simulink model "bh_boat_stabilizer_model"  (R2022b)
settings: Solver=ode15s  StartTime=0.0  StopTime=45  RelTol=1e-6  AbsTol=1e-6  EnableMultiTasking=on
undefined symbols (not defined in the file or in its folder): cage, disk, hull, my_points, sigbuilder_block, stand, X, Y, Z
libraries: sm_lib x37, nesl_utility x18, simulink_extras x18, simulink x1
(part 1 of 3)
settings Model: Creator=bhorton  LastModifiedBy=bhorton
settings SolverCC: ZeroCrossAlgorithm=Adaptive  AlgebraicLoopSolver=TrustRegion
settings DataIOCC: LimitDataPoints=on  MaxDataPoints=10000
settings OptimizationCC: LifeSpan=inf
settings DebuggingCC: UnconnectedInputMsg=warning  UnconnectedOutputMsg=warning  UnconnectedLineMsg=warning  AllowSymbolicDim=off  SFUnexpectedBacktrackingDiag=warning  SFNoUnconditionalDefaultTransitionDiag=warning  SFExecutionAtInitializationDiag=none  SFMachineParentedDataDiag=warning  ArithmeticOperatorsInVariantConditions=warning
settings ModelReferenceCC: EnableRefExpFcnMdlSchedulingChecks=on
settings SFSimCC: SimUseLocalCustomCode=off  CustomCodeUndefinedFunction=UseInterfaceOnly
settings RTWCC: RTWUseLocalCustomCode=off  DLArmComputeVersion=19.05
settings CodeAppCC: StateflowObjectComments=on
settings GRTTargetCC: TargetLangStandard=C89/C90 (ANSI)
settings ConfigComp: CovMetricSettings=dw  CovSaveCumulativeToWorkspaceVar=on  CovSaveSingleToWorkspaceVar=on  CovExternalEMLEnable=off  CovSFcnEnable=off
settings SimscapeCC: SimscapeLogType=all  SimscapeLogSimulationStatistics=on  SimscapeLogDataHistory=10000
settings ExplorerConfigSet: InternalSimMechanicsExplorerSettings="<ExplorerConfiguration><canonicalview>default</canonicalview><AnimationSetting><BasePlaybackSpeed>1.0</BasePlaybackSpeed><PlaybackSpeedFactor>1.0</PlaybackSpeedFactor></AnimationSetting><TilePanel><TileInfo><Tiles Columns=\"2\" Count=\"3\" Rows=\"2\"><Column Weight=\"0.5\"/><Column Weight=\"0.5\"/><Row Weight=\"0.4994\"/><Row Weight=\"0.5006\"/><Tile Height=\"2\" Width=\"1\" X=\"0\" Y=\"0\"/><Tile Height=\"1\" Width=\"1\" X=\"1\" Y=\"0\"/><Tile Height=\"1\" Width=\"1\" X=\"1\" Y=\"1\"/></Tiles></TileInfo><SceneInfo><SceneViewer><BGColor><R>0.60000002384185791</R><G>0.60000002384185791</G><B>0.60000002384185791</B></BGColor><Camera><DoPerspective>off</DoPerspective><Position><X>2.72907980115163751</X><Y>1.63827710737355892</Y><Z>5.84466597133086818</Z></Position><Center><X>1.48957165804863778</X><Y>-0.312477395456248752</Y><Z>2.71114995707715156</Z></Center><Up><X>0.0871556787867786148</X><Y>0.8298702872998307</Y><Z>-0.551107243567087735</Z></Up><ViewLimDist>1</ViewLimDist><YLim>5.28419304463390116</YLim><XLim>3.96508464876347055</XLim></Camera></SceneViewer><SceneViewer><BGColor><R>0.60000002384185791</R><G>0.60000002384185791</G><B>0.60000002384185791</B></BGColor><Camera><DoPerspective>off</DoPerspective><Position><X>0.174100554176560618</X><Y>2.79843990503689621</Y><Z>0.284823193336330216</Z></Position><Center><X>0.177652103694306729</X><Y>-0.924710698878394188</Y><Z>0.283383219246318929</Z></Center><Up><X>0.00583965905908712894</X><Y>0.000392326129121878253</Y><Z>-0.999982872084458463</Z></Up><ViewLimDist>1</ViewLimDist><YLim>0.869664947050413972</YLim><XLim>1.32261544030583789</XLim></Camera></SceneViewer><SceneViewer><BGColor><R>0.60000002384185791</R><G>0.60000002384185791</G><B>0.60000002384185791</B></BGColor><Camera><DoPerspective>off</DoPerspective><Position><X>-0.273643330341835023</X><Y>-1.00050075945724948</Y><Z>3.47750989252231513</Z></Position><Center><X>-0.273643330341835023</X><Y>-1.00050075945724948</Y><Z>-3.69061607941034708e-08</Z></Center><Up><X>0</X><Y>1</Y><Z>-0</Z></Up><ViewLimDist>1</ViewLimDist><YLim>2.77031267511226043</YLim><XLim>4.21318386006656276</XLim></Camera></SceneViewer></SceneInfo></TilePanel><MechEditorPanel><Cameras/><GfxPanelCameraMap/><VideoCreator><PlaybackSpeedRatio>1.0</PlaybackSpeedRatio><FrameRate>30</FrameRate><VideoFormat>Motion JPEG AVI</VideoFormat><FrameSize>auto</FrameSize></VideoCreator></MechEditorPanel></ExplorerConfiguration>"

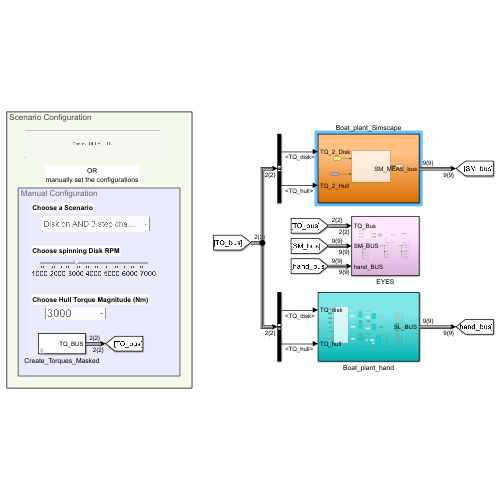
[thumbnail: Simulink's stored preview of the top-level diagram]
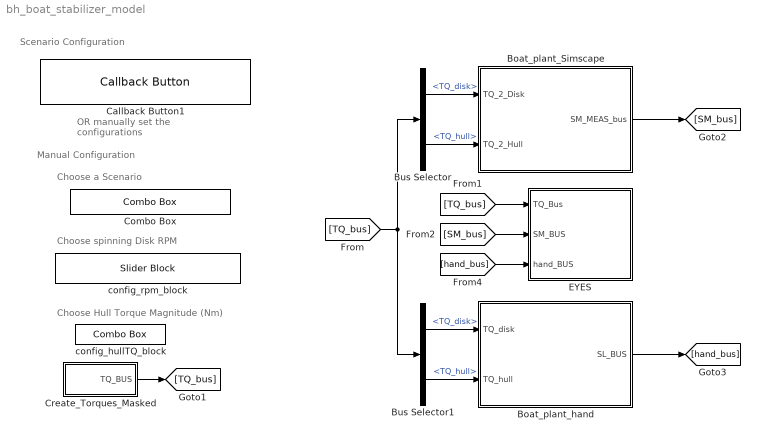
== system bh_boat_stabilizer_model ==
  note: Scenario Configuration
  note: OR
      | manually set the configurations
  note: Choose a Scenario
  note: Manual Configuration
  note: Choose spinning Disk RPM
  note: Choose Hull Torque Magnitude (Nm)
  Boat_plant_Simscape : Subsystem
  Boat_plant_hand : Subsystem
  Bus Selector : BusSelector  OutputSignals=TQ_disk,TQ_hull
  Bus Selector1 : BusSelector  OutputSignals=TQ_disk,TQ_hull
  Callback Button1 : CallbackButton  ButtonText=Choose DEFAULTS
      settings: ClickFcn=|
      | THE_BLOCK = [bdroot, '/Create_Torques_Masked'];
      | 
      | set_param(THE_BLOCK,'the_scenario','1');
      | set_param(THE_BLOCK,'the_disk_rpm','3000');
      | set_param(THE_BLOCK,'the_tau_hull','3000');
  Combo Box : ComboBox  LabelPosition=Hide  SelectedLabel=Disk on AND 3 step changes
      settings: Values={{'NO Stabilization (disk is NOT spinning)', 'Spin up disk BEFORE Disturbance', 'Spin up disk AFTER disturbance', 'Disk always spinning', 'Disk on AND 3 step changes', 'Spin Ramp to 10 percent'}, [1 2 3 4 5 6]}
  Create_Torques_Masked : Subsystem  mask{the_scenario=5, the_disk_rpm=3025.477707006369, the_tau_hull=3000}
      mask prompts: the_scenario "Scenario ID"; the_disk_rpm "Disk RPM"; the_tau_hull "Magnitude of HULL torque (N.m)"
      mask init:
      | THE_BLOCK = [gcb,'/my_sig_builder'];
      | signalbuilder(THE_BLOCK,'activegroup',the_scenario)
  EYES : Subsystem
  config_hullTQ_block : ComboBox  LabelPosition=Hide  SelectedLabel=3000
      settings: Values={{'1000', '3000', '5000', '7000', '9000', '11000'}, [1000 3000 5000 7000 9000 11000]}
  config_rpm_block : SliderBlock  LabelPosition=Hide  ScaleMin=1000  ScaleMax=7000  TickInterval=1000
  wires:
  Bus Selector/1 -> Boat_plant_Simscape/1(TQ_2_Disk)  "<TQ_disk>"
  Bus Selector/2 -> Boat_plant_Simscape/2(TQ_2_Hull)  "<TQ_hull>"
  Boat_plant_Simscape/1(SM_MEAS_bus) -> [SM_bus]
  [SM_bus] -> EYES/2(SM_BUS)
  [TQ_bus] -> EYES/1(TQ_Bus)
  Boat_plant_hand/1(SL_BUS) -> [hand_bus]
  [TQ_bus] -> Bus Selector1/1, Bus Selector/1
  [hand_bus] -> EYES/3(hand_BUS)
  Create_Torques_Masked/1(TQ_BUS) -> [TQ_bus]
  Bus Selector1/1 -> Boat_plant_hand/1(TQ_disk)  "<TQ_disk>"
  Bus Selector1/2 -> Boat_plant_hand/2(TQ_hull)  "<TQ_hull>"

== system bh_boat_stabilizer_model/Boat_plant_Simscape ==
  TQ_2_Disk : Inport
  TQ_2_Hull : Inport  Port=2
  Boat_SM : Subsystem
  SM_MEAS_bus : Outport
  wires:
  TQ_2_Disk/1 -> Boat_SM/1(TQ_spin_disk)
  Boat_SM/1(SM_MEAS_bus) -> SM_MEAS_bus/1
  TQ_2_Hull/1 -> Boat_SM/2(TQ_2_Hull)

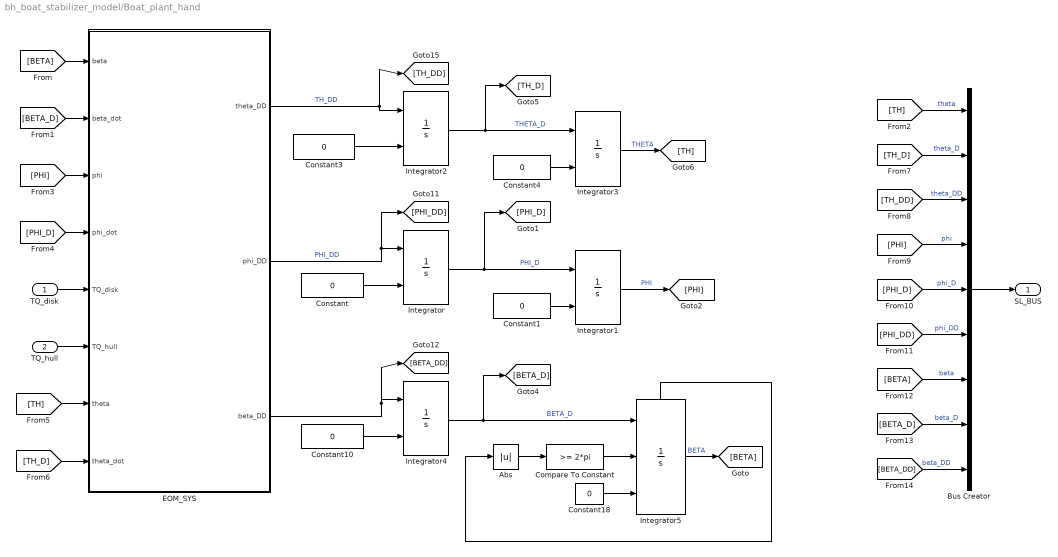
== system bh_boat_stabilizer_model/Boat_plant_hand ==
  TQ_disk : Inport
  TQ_hull : Inport  Port=2
  Abs : Abs  SaturateOnIntegerOverflow=off
  Bus Creator : BusCreator  Inputs=9
  Compare To Constant : simulink/Logic and Bit Operations/Compare To Constant  relop=>=  const=2*pi  OutDataTypeStr=boolean
  Constant{,1,3..4,10,18} (6 alike) : Constant  Value=0
  EOM_SYS : Subsystem
  Integrator{,1..4} (5 alike) : Integrator  InitialConditionSource=external
  Integrator5 : Integrator  ExternalReset=either  InitialConditionSource=external  ShowStatePort=on  AbsoluteTolerance=1e-8
  SL_BUS : Outport
  wires:
  Integrator3/1 -> [TH]  "THETA"
  Integrator4/1 -> [BETA_D], Integrator5/1  "BETA_D"
  Constant4/1 -> Integrator3/2
  Integrator2/1 -> [TH_D], Integrator3/1  "THETA_D"
  Integrator/1 -> [PHI_D], Integrator1/1  "PHI_D"
  Constant18/1 -> Integrator5/3
  Constant1/1 -> Integrator1/2
  Constant10/1 -> Integrator4/2
  Integrator1/1 -> [PHI]  "PHI"
  Constant/1 -> Integrator/2
  Constant3/1 -> Integrator2/2
  Integrator5/1 -> [BETA]  "BETA"
  EOM_SYS/1(theta_DD) -> [TH_DD], Integrator2/1  "TH_DD"
  EOM_SYS/2(phi_DD) -> [PHI_DD], Integrator/1  "PHI_DD"
  EOM_SYS/3(beta_DD) -> [BETA_DD], Integrator4/1
  TQ_disk/1 -> EOM_SYS/5(TQ_disk)
  TQ_hull/1 -> EOM_SYS/6(TQ_hull)
  [BETA_D] -> EOM_SYS/2(beta_dot)
  [BETA] -> EOM_SYS/1(beta)
  [TH_D] -> EOM_SYS/8(theta_dot)
  [TH] -> EOM_SYS/7(theta)
  [PHI_D] -> EOM_SYS/4(phi_dot)
  [PHI] -> EOM_SYS/3(phi)
  Bus Creator/1 -> SL_BUS/1
  [TH] -> Bus Creator/1  "theta"
  [TH_D] -> Bus Creator/2  "theta_D"
  [TH_DD] -> Bus Creator/3  "theta_DD"
  [PHI] -> Bus Creator/4  "phi"
  [PHI_D] -> Bus Creator/5  "phi_D"
  [PHI_DD] -> Bus Creator/6  "phi_DD"
  [BETA_DD] -> Bus Creator/9  "beta_DD"
  [BETA_D] -> Bus Creator/8  "beta_D"
  [BETA] -> Bus Creator/7  "beta"
  Abs/1 -> Compare To Constant/1
  Compare To Constant/1 -> Integrator5/2
  Integrator5/State -> Abs/1

== system bh_boat_stabilizer_model/Create_Torques_Masked ==
  Bus Creator : BusCreator  Inputs=2
  Create_DISK_w_TQ : Subsystem
  Enabled Subsystem1 : Subsystem  TreatAsAtomicUnit=on
  my_sig_builder : Subsystem  Tag=STV Subsys  LoadFcn=sigbuilder_block('load');  StartFcn=sigbuilder_block('start');  StopFcn=sigbuilder_block('stop');  ClipboardFcn=sigbuilder_block('clipboard');  mask(Sigbuilder block){tuvar=[0:10]}
      mask help: Simulink:masks:SigbuilderBlock_MD
      mask init:
      | if ~strcmp(get_param(bdroot(gcbh),'SimulationStatus'),'stopped') tuvar = sigbuilder_block('maskInit'); end
      settings: CopyFcn=sigbuilder_block('copy');  DeleteFcn=sigbuilder_block('delete');  ModelCloseFcn=sigbuilder_block('modelClose');  PreSaveFcn=sigbuilder_block('preSave');  PauseFcn=sigbuilder_block('pause');  ContinueFcn=sigbuilder_block('continue');  NameChangeFcn=sigbuilder_block('namechange');  OpenFcn=sigbuilder_block('open',[437.6 199.2 550.4 400 ]);  CloseFcn=sigbuilder_block('close');
      mask Display: plot(0, 0, 100, 100,[2, 2, 32, 32, 2], [68, 8, 8, 68, 68],[32, 2], [38, 38], [32, 19, 2],[53, 60, 44], [32, 17, 17, 2],[16, 16, 31, 31]);txt = getActiveGroup(gcbh);text(2, 100, txt,'verticalAlignment', 'top');
  TQ_BUS : Outport
  wires:
  my_sig_builder/1(DISK) -> Create_DISK_w_TQ/1(w_disk_normalised)
  Create_DISK_w_TQ/1(TQ) -> Bus Creator/1  "TQ_disk"
  Enabled Subsystem1/1(Out1) -> Bus Creator/2  "TQ_hull"
  my_sig_builder/2(HULL) -> Enabled Subsystem1/Enable
  Bus Creator/1 -> TQ_BUS/1

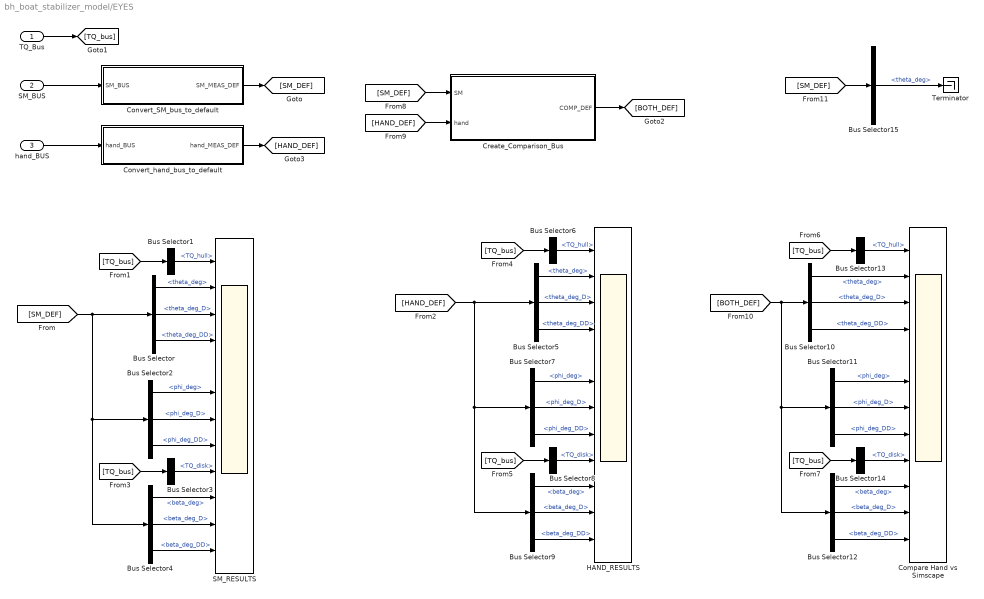
== system bh_boat_stabilizer_model/EYES ==
  TQ_Bus : Inport
  SM_BUS : Inport  Port=2
  hand_BUS : Inport  Port=3
  Bus Selector : BusSelector  OutputSignals=theta_deg,theta_deg_D,theta_deg_DD
  Bus Selector1 : BusSelector  OutputSignals=TQ_hull
  Bus Selector10 : BusSelector  OutputSignals=theta_deg,theta_deg_D,theta_deg_DD
  Bus Selector11 : BusSelector  OutputSignals=phi_deg,phi_deg_D,phi_deg_DD
  Bus Selector12 : BusSelector  OutputSignals=beta_deg,beta_deg_D,beta_deg_DD
  Bus Selector13 : BusSelector  OutputSignals=TQ_hull
  Bus Selector14 : BusSelector  OutputSignals=TQ_disk
  Bus Selector15 : BusSelector  OutputSignals=theta_deg
  Bus Selector2 : BusSelector  OutputSignals=phi_deg,phi_deg_D,phi_deg_DD
  Bus Selector3 : BusSelector  OutputSignals=TQ_disk
  Bus Selector4 : BusSelector  OutputSignals=beta_deg,beta_deg_D,beta_deg_DD
  Bus Selector5 : BusSelector  OutputSignals=theta_deg,theta_deg_D,theta_deg_DD
  Bus Selector6 : BusSelector  OutputSignals=TQ_hull
  Bus Selector7 : BusSelector  OutputSignals=phi_deg,phi_deg_D,phi_deg_DD
  Bus Selector8 : BusSelector  OutputSignals=TQ_disk
  Bus Selector9 : BusSelector  OutputSignals=beta_deg,beta_deg_D,beta_deg_DD
  Compare Hand vs Simscape : Scope  NumInputPorts=12
  Convert_SM_bus_to_default : Subsystem
  Convert_hand_bus_to_default : Subsystem
  Create_Comparison_Bus : Subsystem
  HAND_RESULTS : Scope  NumInputPorts=12
  SM_RESULTS : Scope  NumInputPorts=12
  Terminator : Terminator
  wires:
  SM_BUS/1 -> Convert_SM_bus_to_default/1(SM_BUS)
  Convert_SM_bus_to_default/1(SM_MEAS_DEF) -> [SM_DEF]
  TQ_Bus/1 -> [TQ_bus]
  [TQ_bus] -> Bus Selector1/1
  Bus Selector1/1 -> SM_RESULTS/1  "<TQ_hull>"
  Bus Selector/1 -> SM_RESULTS/2  "<theta_deg>"
  Bus Selector/3 -> SM_RESULTS/4  "<theta_deg_DD>"
  Bus Selector/2 -> SM_RESULTS/3  "<theta_deg_D>"
  Bus Selector2/1 -> SM_RESULTS/6  "<phi_deg>"
  Bus Selector2/2 -> SM_RESULTS/7  "<phi_deg_D>"
  Bus Selector2/3 -> SM_RESULTS/8  "<phi_deg_DD>"
  [TQ_bus] -> Bus Selector3/1
  Bus Selector3/1 -> SM_RESULTS/9  "<TQ_disk>"
  [SM_DEF] -> Bus Selector2/1, Bus Selector4/1, Bus Selector/1
  Bus Selector4/1 -> SM_RESULTS/10  "<beta_deg>"
  Bus Selector4/2 -> SM_RESULTS/11  "<beta_deg_D>"
  Bus Selector4/3 -> SM_RESULTS/12  "<beta_deg_DD>"
  hand_BUS/1 -> Convert_hand_bus_to_default/1(hand_BUS)
  Convert_hand_bus_to_default/1(hand_MEAS_DEF) -> [HAND_DEF]
  Bus Selector9/2 -> HAND_RESULTS/11  "<beta_deg_D>"
  Bus Selector9/3 -> HAND_RESULTS/12  "<beta_deg_DD>"
  Bus Selector7/1 -> HAND_RESULTS/6  "<phi_deg>"
  Bus Selector6/1 -> HAND_RESULTS/1  "<TQ_hull>"
  Bus Selector7/2 -> HAND_RESULTS/7  "<phi_deg_D>"
  [TQ_bus] -> Bus Selector6/1
  Bus Selector5/1 -> HAND_RESULTS/2  "<theta_deg>"
  [TQ_bus] -> Bus Selector8/1
  Bus Selector8/1 -> HAND_RESULTS/9  "<TQ_disk>"
  Bus Selector5/2 -> HAND_RESULTS/3  "<theta_deg_D>"
  [HAND_DEF] -> Bus Selector7/1, Bus Selector9/1, Bus Selector5/1
  Bus Selector9/1 -> HAND_RESULTS/10  "<beta_deg>"
  Bus Selector7/3 -> HAND_RESULTS/8  "<phi_deg_DD>"
  Bus Selector5/3 -> HAND_RESULTS/4  "<theta_deg_DD>"
  Bus Selector10/1 -> Compare Hand vs Simscape/2  "<theta_deg>"
  Bus Selector10/2 -> Compare Hand vs Simscape/3  "<theta_deg_D>"
  Bus Selector10/3 -> Compare Hand vs Simscape/4  "<theta_deg_DD>"
  [HAND_DEF] -> Create_Comparison_Bus/2(hand)
  [SM_DEF] -> Create_Comparison_Bus/1(SM)
  Create_Comparison_Bus/1(COMP_DEF) -> [BOTH_DEF]
  [BOTH_DEF] -> Bus Selector12/1, Bus Selector11/1, Bus Selector10/1
  Bus Selector12/1 -> Compare Hand vs Simscape/10  "<beta_deg>"
  Bus Selector12/2 -> Compare Hand vs Simscape/11  "<beta_deg_D>"
  Bus Selector12/3 -> Compare Hand vs Simscape/12  "<beta_deg_DD>"
  Bus Selector11/1 -> Compare Hand vs Simscape/6  "<phi_deg>"
  Bus Selector11/2 -> Compare Hand vs Simscape/7  "<phi_deg_D>"
  Bus Selector11/3 -> Compare Hand vs Simscape/8  "<phi_deg_DD>"
  Bus Selector13/1 -> Compare Hand vs Simscape/1  "<TQ_hull>"
  [TQ_bus] -> Bus Selector13/1
  [TQ_bus] -> Bus Selector14/1
  Bus Selector14/1 -> Compare Hand vs Simscape/9  "<TQ_disk>"
  [SM_DEF] -> Bus Selector15/1
  Bus Selector15/1 -> Terminator/1  "<theta_deg>"

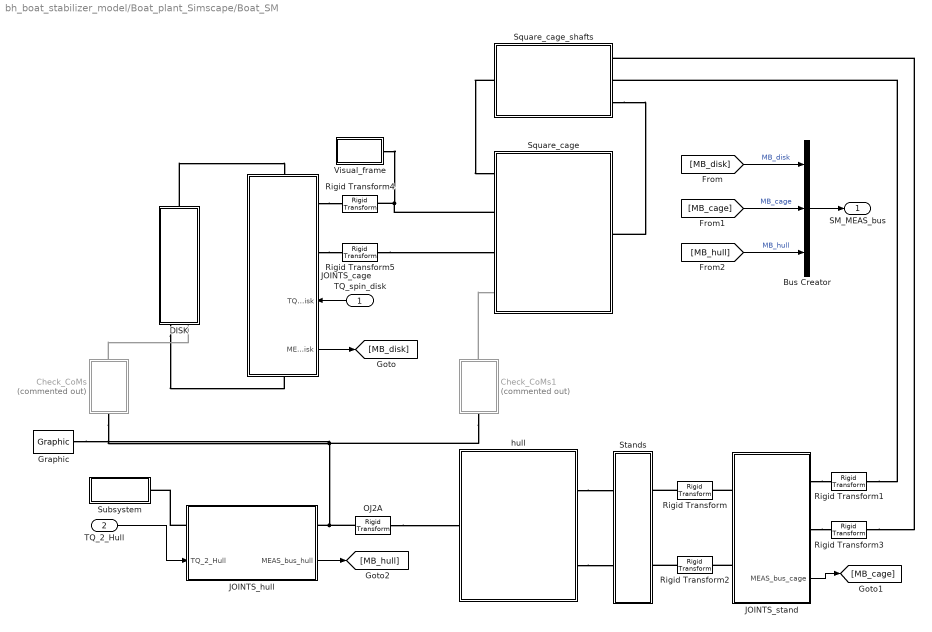
== system bh_boat_stabilizer_model/Boat_plant_Simscape/Boat_SM ==
  TQ_spin_disk : Inport
  TQ_2_Hull : Inport  Port=2
  Bus Creator : BusCreator  Inputs=3
  Check_CoMs : Subsystem  Commented=on
      settings: PortSchema="{\"entries\":[{\"content\":{\"sides\":[{\"content\":{\"connectorIds\":[]},\"type\":\"ConnectorPlacement.EquallySpacedRectSide\",\"uuid\":\"8ed19b4e-1183-4e07-bf69-d3669f8bd5cb\"},{\"content\":{\"connectorIds\":[],\"side\":\"RIGHT\"},\"type\":\"ConnectorPlacement.EquallySpacedRectSide\",\"uuid\":\"73952c4f-7d1b-4c69-9603-d3eee881218d\"},{\"content\":{\"connectorIds\":[\"LConn1\"],\"side\":\"TOP\"},\"type\":\"ConnectorPlacement.EquallySpacedRectSide\",\"uuid\":\"77bc43cc-06ea-441c-8da5-d3750df69a68\"},{\"content\":{\"connectorIds\":[\"RConn1\"],\"side\":\"BOTTOM\"},\"type\":\"ConnectorPlacement.EquallySpacedRectSide\",\"uuid\":\"9e044842-34cb-487c-aed5-c5c152a9fa85\"}]},\"type\":\"ConnectorPlacement.EquallySpacedConnector\",\"uuid\":\"cc47beea-0fb2-477b-9821-656a15c7a45c\"}],\"packageUris\":[\"http://schema.mathworks.com/mf0/Connector/19700101\"],\"version\":\"1.0\"}"
  Check_CoMs1 : Subsystem  Commented=on
      settings: PortSchema="{\"entries\":[{\"content\":{\"sides\":[{\"content\":{\"connectorIds\":[]},\"type\":\"ConnectorPlacement.EquallySpacedRectSide\",\"uuid\":\"8ed19b4e-1183-4e07-bf69-d3669f8bd5cb\"},{\"content\":{\"connectorIds\":[],\"side\":\"RIGHT\"},\"type\":\"ConnectorPlacement.EquallySpacedRectSide\",\"uuid\":\"73952c4f-7d1b-4c69-9603-d3eee881218d\"},{\"content\":{\"connectorIds\":[\"LConn1\"],\"side\":\"TOP\"},\"type\":\"ConnectorPlacement.EquallySpacedRectSide\",\"uuid\":\"77bc43cc-06ea-441c-8da5-d3750df69a68\"},{\"content\":{\"connectorIds\":[\"RConn1\"],\"side\":\"BOTTOM\"},\"type\":\"ConnectorPlacement.EquallySpacedRectSide\",\"uuid\":\"9e044842-34cb-487c-aed5-c5c152a9fa85\"}]},\"type\":\"ConnectorPlacement.EquallySpacedConnector\",\"uuid\":\"cc47beea-0fb2-477b-9821-656a15c7a45c\"}],\"packageUris\":[\"http://schema.mathworks.com/mf0/Connector/19700101\"],\"version\":\"1.0\"}"
  DISK : Subsystem  mask{D_shaft=disk.shaft_D, L_shaft=disk.shaft_L, density_shaft=disk.shaft_density, D_disk=disk.D, L_disk=disk.L, density=disk.density}
      mask prompts: D_shaft "Shaft diam (m)"; L_shaft "Shaft Length (m)"; density_shaft "Shaft density (kg/m^3)"; D_disk "Disk diam (m)"; L_disk "Disk Length (m)"; density "Disk density (kg/m^3)"
  Graphic : sm_lib/Body Elements/Graphic  GraphicType=Marker  MarkerShape=Frame  MarkerSize=40  GraphicVisPropType=SimpleVisualProperties  GraphicDiffuseColor=[0.4 0.4 1.0]  GraphicSpecularColor=[0.5 0.5 0.5 1.0]  GraphicAmbientColor=[0.15 0.15 0.15 1.0]  GraphicEmissiveColor=[0.0 0.0 0.0 1.0]  GraphicShininess=75  GraphicOpacity=1.0
  JOINTS_cage : Subsystem
      settings: PortSchema="{\"entries\":[{\"content\":{\"sides\":[{\"content\":{\"connectorIds\":[]},\"type\":\"ConnectorPlacement.EquallySpacedRectSide\",\"uuid\":\"be4d2694-6a62-440c-90ae-db4dffa0fd3a\"},{\"content\":{\"connectorIds\":[\"RConn1\",\"RConn2\",\"In1\",\"Out1\"],\"side\":\"RIGHT\"},\"type\":\"ConnectorPlacement.EquallySpacedRectSide\",\"uuid\":\"ab45e458-13ad-44f6-9477-3131c41a1440\"},{\"content\":{\"connectorIds\":[\"LConn1\"],\"side\":\"TOP\"},\"type\":\"ConnectorPlacement.EquallySpacedRectSide\",\"uuid\":\"f5a3ad65-3a41-4ce7-9c2f-251303d2413e\"},{\"content\":{\"connectorIds\":[\"RConn3\"],\"side\":\"BOTTOM\"},\"type\":\"ConnectorPlacement.EquallySpacedRectSide\",\"uuid\":\"5613cf96-304b-49cb-813b-3f7d46593de8\"}]},\"type\":\"ConnectorPlacement.EquallySpacedConnector\",\"uuid\":\"b705f2a7-e9ac-4d64-aa26-3dc8e599ccc9\"}],\"packageUris\":[\"http://schema.mathworks.com/mf0/Connector/19700101\"],\"version\":\"1.0\"}"
  JOINTS_hull : Subsystem
      settings: PortSchema="{\"entries\":[{\"content\":{\"sides\":[{\"content\":{\"connectorIds\":[\"LConn1\",\"In1\"]},\"type\":\"ConnectorPlacement.EquallySpacedRectSide\",\"uuid\":\"e5f6a5c8-9e7e-4d4f-a156-8d2f522016b6\"},{\"content\":{\"connectorIds\":[\"RConn1\",\"Out1\"],\"side\":\"RIGHT\"},\"type\":\"ConnectorPlacement.EquallySpacedRectSide\",\"uuid\":\"d52b2acd-f075-4b35-bae2-891ffaf718b5\"},{\"content\":{\"connectorIds\":[],\"side\":\"TOP\"},\"type\":\"ConnectorPlacement.EquallySpacedRectSide\",\"uuid\":\"04e03750-ca17-4a1e-8c88-a8877bdd9a93\"}]},\"type\":\"ConnectorPlacement.EquallySpacedConnector\",\"uuid\":\"a354eef0-eda7-4596-be43-d923e734c9ea\"}],\"packageUris\":[\"http://schema.mathworks.com/mf0/Connector/19700101\"],\"version\":\"1.0\"}"
  JOINTS_stand : Subsystem
      settings: PortSchema="{\"entries\":[{\"content\":{\"sides\":[{\"content\":{\"connectorIds\":[\"LConn1\",\"LConn2\"]},\"type\":\"ConnectorPlacement.EquallySpacedRectSide\",\"uuid\":\"d8290ed1-c238-4653-a380-fe4cd0d1c1d6\"},{\"content\":{\"connectorIds\":[\"RConn1\",\"RConn2\",\"Out1\"],\"side\":\"RIGHT\"},\"type\":\"ConnectorPlacement.EquallySpacedRectSide\",\"uuid\":\"362a6e20-25d8-44a0-b01e-70408c158174\"},{\"content\":{\"connectorIds\":[],\"side\":\"TOP\"},\"type\":\"ConnectorPlacement.EquallySpacedRectSide\",\"uuid\":\"83d9be7d-8ddb-4200-9f05-eb3df9a34d4e\"}]},\"type\":\"ConnectorPlacement.EquallySpacedConnector\",\"uuid\":\"234fcb63-a29e-49fe-b79c-37e2d67e369e\"}],\"packageUris\":[\"http://schema.mathworks.com/mf0/Connector/19700101\"],\"version\":\"1.0\"}"
  OJ2A : sm_lib/Frames and Transforms/Rigid Transform  TranslationMethod=Cartesian  TranslationStandardOffset=0  TranslationLengthUnit=m  TranslationStandardAxis=+Z  TranslationCartesianOffset=my_points.A_rel2O  TranslationROffset=0  TranslationROffsetUnits=m  TranslationZOffset=0  TranslationZOffsetUnits=m  TranslationThetaOffset=0  TranslationThetaOffsetUnits=deg  RotationMethod=None  RotationAngleUnits=deg  RotationStandardAxis=+Z  RotationAngle=0.0  RotationArbitraryAxis=[0 0 1]  FollAlignAxisA=+Z  BaseAlignAxisA=+Y  FollAlignAxisB=+X  BaseAlignAxisB=+X  RotationSequenceAxes=FollowerAxes  RotationSequence=XYX  RotationSequenceAngles=[0 0 0]  RotationSequenceAnglesUnits=deg  RotationMatrix=[1 0 0; 0 1 0; 0 0 1]  Quaternion=[1 0 0 0]
  Rigid Transform : sm_lib/Frames and Transforms/Rigid Transform  TranslationMethod=None  TranslationStandardOffset=0  TranslationLengthUnit=m  TranslationStandardAxis=+Z  TranslationCartesianOffset=[0 0 0]  TranslationROffset=0  TranslationROffsetUnits=m  TranslationZOffset=0  TranslationZOffsetUnits=m  TranslationThetaOffset=0  TranslationThetaOffsetUnits=deg  RotationMethod=AlignedAxes  RotationAngleUnits=deg  RotationStandardAxis=+Z  RotationAngle=0.0  RotationArbitraryAxis=[0 0 1]  FollAlignAxisA=+Z  BaseAlignAxisA=+X  FollAlignAxisB=+Y  BaseAlignAxisB=+Y  RotationSequenceAxes=FollowerAxes  RotationSequence=XYX  RotationSequenceAngles=[0 0 0]  RotationSequenceAnglesUnits=deg  RotationMatrix=[1 0 0; 0 1 0; 0 0 1]  Quaternion=[1 0 0 0]
  Rigid Transform1 : sm_lib/Frames and Transforms/Rigid Transform  TranslationMethod=None  TranslationStandardOffset=0  TranslationLengthUnit=m  TranslationStandardAxis=+Z  TranslationCartesianOffset=[0 0 0]  TranslationROffset=0  TranslationROffsetUnits=m  TranslationZOffset=0  TranslationZOffsetUnits=m  TranslationThetaOffset=0  TranslationThetaOffsetUnits=deg  RotationMethod=AlignedAxes  RotationAngleUnits=deg  RotationStandardAxis=+Z  RotationAngle=0.0  RotationArbitraryAxis=[0 0 1]  FollAlignAxisA=+X  BaseAlignAxisA=+Z  FollAlignAxisB=+Y  BaseAlignAxisB=+Y  RotationSequenceAxes=FollowerAxes  RotationSequence=XYX  RotationSequenceAngles=[0 0 0]  RotationSequenceAnglesUnits=deg  RotationMatrix=[1 0 0; 0 1 0; 0 0 1]  Quaternion=[1 0 0 0]
  Rigid Transform2 : sm_lib/Frames and Transforms/Rigid Transform  TranslationMethod=None  TranslationStandardOffset=0  TranslationLengthUnit=m  TranslationStandardAxis=+Z  TranslationCartesianOffset=[0 0 0]  TranslationROffset=0  TranslationROffsetUnits=m  TranslationZOffset=0  TranslationZOffsetUnits=m  TranslationThetaOffset=0  TranslationThetaOffsetUnits=deg  RotationMethod=AlignedAxes  RotationAngleUnits=deg  RotationStandardAxis=+Z  RotationAngle=0.0  RotationArbitraryAxis=[0 0 1]  FollAlignAxisA=+Z  BaseAlignAxisA=+X  FollAlignAxisB=+Y  BaseAlignAxisB=+Y  RotationSequenceAxes=FollowerAxes  RotationSequence=XYX  RotationSequenceAngles=[0 0 0]  RotationSequenceAnglesUnits=deg  RotationMatrix=[1 0 0; 0 1 0; 0 0 1]  Quaternion=[1 0 0 0]
  Rigid Transform3 : sm_lib/Frames and Transforms/Rigid Transform  TranslationMethod=None  TranslationStandardOffset=0  TranslationLengthUnit=m  TranslationStandardAxis=+Z  TranslationCartesianOffset=[0 0 0]  TranslationROffset=0  TranslationROffsetUnits=m  TranslationZOffset=0  TranslationZOffsetUnits=m  TranslationThetaOffset=0  TranslationThetaOffsetUnits=deg  RotationMethod=AlignedAxes  RotationAngleUnits=deg  RotationStandardAxis=+Z  RotationAngle=0.0  RotationArbitraryAxis=[0 0 1]  FollAlignAxisA=+X  BaseAlignAxisA=+Z  FollAlignAxisB=+Y  BaseAlignAxisB=+Y  RotationSequenceAxes=FollowerAxes  RotationSequence=XYX  RotationSequenceAngles=[0 0 0]  RotationSequenceAnglesUnits=deg  RotationMatrix=[1 0 0; 0 1 0; 0 0 1]  Quaternion=[1 0 0 0]
  Rigid Transform4 : sm_lib/Frames and Transforms/Rigid Transform  TranslationMethod=None  TranslationStandardOffset=0  TranslationLengthUnit=m  TranslationStandardAxis=+Z  TranslationCartesianOffset=[0 0 0]  TranslationROffset=0  TranslationROffsetUnits=m  TranslationZOffset=0  TranslationZOffsetUnits=m  TranslationThetaOffset=0  TranslationThetaOffsetUnits=deg  RotationMethod=AlignedAxes  RotationAngleUnits=deg  RotationStandardAxis=+Z  RotationAngle=0.0  RotationArbitraryAxis=[0 0 1]  FollAlignAxisA=+Z  BaseAlignAxisA=+Y  FollAlignAxisB=+X  BaseAlignAxisB=+X  RotationSequenceAxes=FollowerAxes  RotationSequence=XYX  RotationSequenceAngles=[0 0 0]  RotationSequenceAnglesUnits=deg  RotationMatrix=[1 0 0; 0 1 0; 0 0 1]  Quaternion=[1 0 0 0]
  Rigid Transform5 : sm_lib/Frames and Transforms/Rigid Transform  TranslationMethod=None  TranslationStandardOffset=0  TranslationLengthUnit=m  TranslationStandardAxis=+Z  TranslationCartesianOffset=[0 0 0]  TranslationROffset=0  TranslationROffsetUnits=m  TranslationZOffset=0  TranslationZOffsetUnits=m  TranslationThetaOffset=0  TranslationThetaOffsetUnits=deg  RotationMethod=AlignedAxes  RotationAngleUnits=deg  RotationStandardAxis=+Z  RotationAngle=0.0  RotationArbitraryAxis=[0 0 1]  FollAlignAxisA=+Z  BaseAlignAxisA=+Y  FollAlignAxisB=+X  BaseAlignAxisB=+X  RotationSequenceAxes=FollowerAxes  RotationSequence=XYX  RotationSequenceAngles=[0 0 0]  RotationSequenceAnglesUnits=deg  RotationMatrix=[1 0 0; 0 1 0; 0 0 1]  Quaternion=[1 0 0 0]
  Square_cage : Subsystem  mask{Lx=cage.Lx, Ly=cage.Ly, tx=cage.tx, ty=cage.ty, tz=cage.tz, density=cage.density}
      mask prompts: Lx "Length_X  (m)"; Ly "Length_Y  (m)"; tx "tx  (m)"; ty "ty  (m)"; tz "tz (m)"; density "density (kg/m3)"
      mask init:
      | OBJ = bh_cage_CLS(Lx,Ly,tx,ty);
  Square_cage_shafts : Subsystem  mask{L_rx=cage.L_rx, D=cage.D, density=cage.density}
      mask prompts: density "density (kg/m3)"
  Stands : Subsystem  mask{Ly=stand.Ly, tx=stand.tx, tz=stand.tz, density=stand.density}
      mask prompts: Ly "Ly (m)"; tx "tx (m)"; tz "tz (m)"; density "density (kg/m^3)"
  Subsystem : Subsystem
  Visual_frame : Subsystem
  hull : Subsystem  mask{Lix=hull.L_ix, Liy=hull.L_iy, tx=hull.tx, ty=hull.ty, tz=hull.tz, density=hull.density, posBrel2A=my_points.B_rel2A, posCrel2A=my_points.C_rel2A}
      mask prompts: Lix "Length_iX  (m)"; Liy "Length_iY  (m)"; tx "tx  (m)"; ty "ty  (m)"; tz "tz (m)"; density "density (kg/m3)"; posBrel2A "Position_B relative to A (m)"; posCrel2A "Position_C relative to A (m)"
      mask init:
      | OBJ = bh_hull_CLS(Lix,Liy,tx,ty);
  SM_MEAS_bus : Outport
  wires:
  TQ_spin_disk/1 -> JOINTS_cage/1(TQ_spin_disk)
  JOINTS_stand/1(MEAS_bus_cage) -> [MB_cage]
  JOINTS_cage/1(MEAS_bus_disk) -> [MB_disk]
  [MB_cage] -> Bus Creator/2  "MB_cage"
  [MB_disk] -> Bus Creator/1  "MB_disk"
  Bus Creator/1 -> SM_MEAS_bus/1
  TQ_2_Hull/1 -> JOINTS_hull/1(TQ_2_Hull)
  JOINTS_hull/1(MEAS_bus_hull) -> [MB_hull]
  [MB_hull] -> Bus Creator/3  "MB_hull"
  connections:
  Square_cage/LConn2 -- Visual_frame/RConn1 -- Rigid Transform4/LConn1
  Rigid Transform3/RConn1 -- Square_cage_shafts/RConn1
  hull/RConn2 -- Stands/RConn2
  hull/RConn1 -- Stands/RConn1
  Rigid Transform/LConn1 -- Stands/LConn1
  Rigid Transform1/RConn1 -- Square_cage_shafts/RConn2
  Square_cage_shafts/LConn1 -- Square_cage/LConn1
  Rigid Transform2/LConn1 -- Stands/LConn2
  Rigid Transform5/LConn1 -- Square_cage/LConn3
  Square_cage_shafts/RConn3 -- Square_cage/RConn1
  OJ2A/RConn1 -- hull/LConn2
  JOINTS_stand/RConn2 -- Rigid Transform3/LConn1
  JOINTS_stand/RConn1 -- Rigid Transform1/LConn1
  JOINTS_stand/LConn1 -- Rigid Transform/RConn1
  JOINTS_stand/LConn2 -- Rigid Transform2/RConn1
  JOINTS_cage/RConn1 -- Rigid Transform4/RConn1
  JOINTS_cage/RConn2 -- Rigid Transform5/RConn1
  DISK/RConn1 -- JOINTS_cage/LConn1
  DISK/LConn1 -- JOINTS_cage/RConn3
  JOINTS_hull/LConn1 -- Subsystem/RConn1
  OJ2A/LConn1 -- Check_CoMs1/RConn1 -- Graphic/RConn1 -- Check_CoMs/RConn1 -- JOINTS_hull/RConn1
  Check_CoMs/LConn1 -- DISK/LConn2
  Check_CoMs1/LConn1 -- Square_cage/LConn4

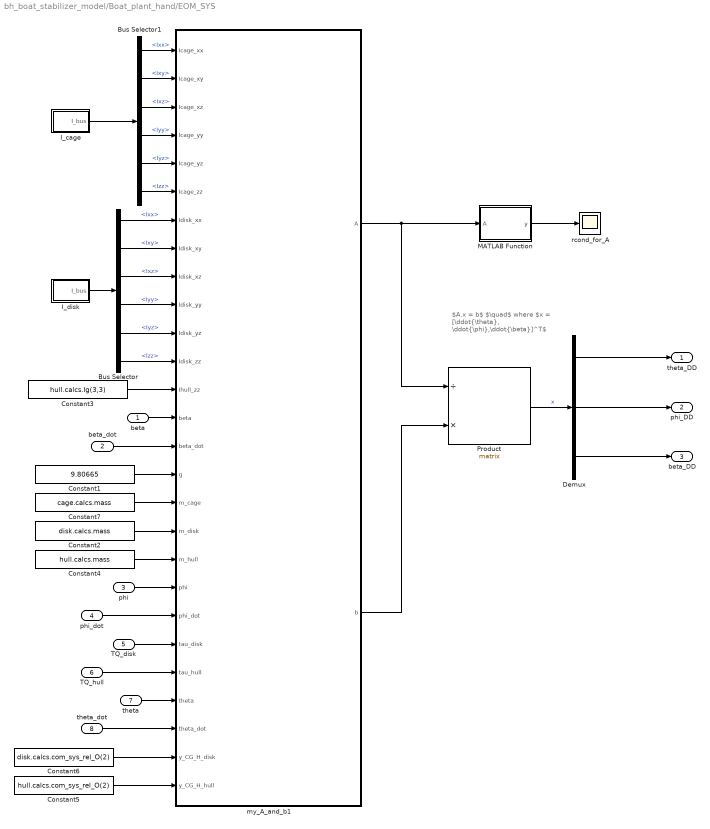
== system bh_boat_stabilizer_model/Boat_plant_hand/EOM_SYS ==
  note: $A.x = b$ $\quad$ where
      |
      | $x = [\ddot{\theta}, \ddot{\phi},\ddot{\beta}]^T$
  beta : Inport
  beta_dot : Inport  Port=2
  phi : Inport  Port=3
  phi_dot : Inport  Port=4
  TQ_disk : Inport  Port=5
  TQ_hull : Inport  Port=6
  theta : Inport  Port=7
  theta_dot : Inport  Port=8
  Bus Selector : BusSelector  OutputSignals=Ixx,Ixy,Ixz,Iyy,Iyz,Izz
  Bus Selector1 : BusSelector  OutputSignals=Ixx,Ixy,Ixz,Iyy,Iyz,Izz
  Constant1 : Constant  Value=9.80665
  Constant2 : Constant  Value=disk.calcs.mass
  Constant3 : Constant  Value=hull.calcs.Ig(3,3)
  Constant4 : Constant  Value=hull.calcs.mass
  Constant5 : Constant  Value=hull.calcs.com_sys_rel_O(2)
  Constant6 : Constant  Value=disk.calcs.com_sys_rel_O(2)
  Constant7 : Constant  Value=cage.calcs.mass
  Demux : Demux  Outputs=3
  I_cage : Subsystem
  I_disk : Subsystem
  MATLAB Function : MATLAB Function  TreatAsAtomicUnit=on
  Product : Product  Inputs=/*  Multiplication=Matrix(*)
  my_A_and_b1 : MATLAB Function  TreatAsAtomicUnit=on
  rcond_for_A : Scope
  theta_DD : Outport
  phi_DD : Outport  Port=2
  beta_DD : Outport  Port=3
  wires:
  Product/1 -> Demux/1  "x"
  I_disk/1(I_bus) -> Bus Selector/1
  Demux/1 -> theta_DD/1
  Demux/3 -> beta_DD/1
  Demux/2 -> phi_DD/1
  my_A_and_b1/1(A) -> MATLAB Function/1(A), Product/1
  my_A_and_b1/2(b) -> Product/2
  Bus Selector1/1 -> my_A_and_b1/1(Icage_xx)  "<Ixx>"
  Bus Selector1/2 -> my_A_and_b1/2(Icage_xy)  "<Ixy>"
  Bus Selector1/3 -> my_A_and_b1/3(Icage_xz)  "<Ixz>"
  Bus Selector1/4 -> my_A_and_b1/4(Icage_yy)  "<Iyy>"
  Bus Selector1/5 -> my_A_and_b1/5(Icage_yz)  "<Iyz>"
  Bus Selector1/6 -> my_A_and_b1/6(Icage_zz)  "<Izz>"
  I_cage/1(I_bus) -> Bus Selector1/1
  Bus Selector/1 -> my_A_and_b1/7(Idisk_xx)  "<Ixx>"
  Bus Selector/2 -> my_A_and_b1/8(Idisk_xy)  "<Ixy>"
  Bus Selector/3 -> my_A_and_b1/9(Idisk_xz)  "<Ixz>"
  Bus Selector/4 -> my_A_and_b1/10(Idisk_yy)  "<Iyy>"
  Bus Selector/5 -> my_A_and_b1/11(Idisk_yz)  "<Iyz>"
  Bus Selector/6 -> my_A_and_b1/12(Idisk_zz)  "<Izz>"
  Constant3/1 -> my_A_and_b1/13(Ihull_zz)
  Constant4/1 -> my_A_and_b1/19(m_hull)
  Constant2/1 -> my_A_and_b1/18(m_disk)
  Constant1/1 -> my_A_and_b1/16(g)
  Constant7/1 -> my_A_and_b1/17(m_cage)
  Constant6/1 -> my_A_and_b1/26(y_CG_H_disk)
  Constant5/1 -> my_A_and_b1/27(y_CG_H_hull)
  phi/1 -> my_A_and_b1/20(phi)
  phi_dot/1 -> my_A_and_b1/21(phi_dot)
  TQ_disk/1 -> my_A_and_b1/22(tau_disk)
  TQ_hull/1 -> my_A_and_b1/23(tau_hull)
  theta/1 -> my_A_and_b1/24(theta)
  theta_dot/1 -> my_A_and_b1/25(theta_dot)
  beta/1 -> my_A_and_b1/14(beta)
  beta_dot/1 -> my_A_and_b1/15(beta_dot)
  MATLAB Function/1(y) -> rcond_for_A/1

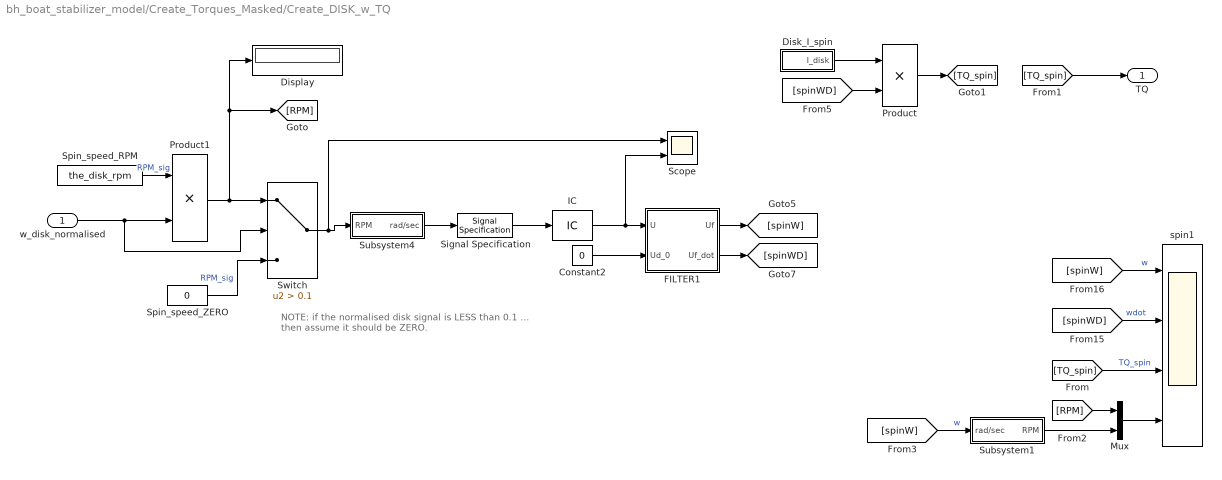
== system bh_boat_stabilizer_model/Create_Torques_Masked/Create_DISK_w_TQ ==
  note: NOTE:  if the normalised disk signal
      | is LESS than 0.1 ... then assume it should be ZERO.
  w_disk_normalised : Inport
  Constant2 : Constant  Value=0
  Disk_I_spin : Subsystem
  Display : Display
  FILTER1 : Subsystem
  IC : InitialCondition  Value=0
  Mux : Mux  Inputs=2
  Product : Product
  Product1 : Product
  Scope : Scope  NumInputPorts=2
  Signal Specification : SignalSpecification  SampleTime=0
  Spin_speed_RPM : Constant  Value=the_disk_rpm
  Spin_speed_ZERO : Constant  Value=0
  Subsystem1 : Subsystem
  Subsystem4 : Subsystem
  Switch : Switch  Criteria=u2 > Threshold  Threshold=0.1  SaturateOnIntegerOverflow=off  InputSameDT=off
  spin1 : Scope  NumInputPorts=4
  TQ : Outport
  wires:
  [spinW] -> spin1/1  "w"
  Product/1 -> [TQ_spin]
  Disk_I_spin/1(I_disk) -> Product/1
  [spinWD] -> Product/2
  [spinWD] -> spin1/2  "wdot"
  Constant2/1 -> FILTER1/2(Ud_0)
  FILTER1/1(Uf) -> [spinW]
  FILTER1/2(Uf_dot) -> [spinWD]
  Switch/1 -> Scope/1, Subsystem4/1(RPM)
  [TQ_spin] -> spin1/3  "TQ_spin"
  [TQ_spin] -> TQ/1
  Spin_speed_ZERO/1 -> Switch/3  "RPM_sig"
  IC/1 -> Scope/2, FILTER1/1(U)
  Subsystem4/1(rad/sec) -> Signal Specification/1
  Signal Specification/1 -> IC/1
  Mux/1 -> spin1/4
  [RPM] -> Mux/1
  [spinW] -> Subsystem1/1(rad/sec)  "w"
  Subsystem1/1(RPM) -> Mux/2
  w_disk_normalised/1 -> Switch/2, Product1/2
  Spin_speed_RPM/1 -> Product1/1  "RPM_sig"
  Product1/1 -> Switch/1, [RPM], Display/1

== system bh_boat_stabilizer_model/Create_Torques_Masked/Enabled Subsystem1 ==
  Enable : EnablePort  StatesWhenEnabling=reset
  Clock : Clock
  Constant : Constant  Value=2*pi
  Constant1 : Constant  Value=0.5
  Constant2 : Constant  Value=the_tau_hull
  Display : Display
  Product : Product
  Product1 : Product
  Product2 : Product
  Trigonometric Function : Trigonometry
  Out1 : Outport  InitialOutput=0
  wires:
  Product/1 -> Trigonometric Function/1
  Constant1/1 -> Product1/2  "f_hz"
  Product2/1 -> Out1/1
  Constant/1 -> Product1/1  "2_PI"
  Clock/1 -> Product/1
  Product1/1 -> Product/2  "w"
  Trigonometric Function/1 -> Product2/1
  Constant2/1 -> Display/1, Product2/2

== system bh_boat_stabilizer_model/Create_Torques_Masked/my_sig_builder ==
  Demux : Demux  Tag=STV Demux  Outputs=2
      settings: DisplayOption=none
  FromWs : FromWorkspace  Tag=STV FromWs  VariableName=tuvar
      SigBuilderData=|
      | common.afterFinalStr = 'Extrapolate'
      | common.sampleTime = 0
      | dataSet(1).timeRange = [0 60]
      | dataSet(1).name = 'NO_STABILIZATION'
      | dataSet(2).timeRange = [0 60]
      | dataSet(2).name = 'DISK_THEN_LOAD'
      | dataSet(3).timeRange = [0 60]
      | dataSet(3).name = 'LOAD_THEN_DISK'
      | dataSet(4).timeRange = [0 60]
      | dataSet(4).name = 'DISK_THEN_LOAD_V2'
      | dataSet(5).timeRange = [0 60]
      | dataSet(5).name = 'DISK_ON_AND_3_STEP_CHANGES'
      | dataSet(6).timeRange = [0 60]
      | dataSet(6).name = 'RAMP_TO_10PC'
      | sbobj.Groups(1).Name = 'NO_STABILIZATION'
      | sbobj.Groups(1).Signals(1).Name = 'DISK'
      | sbobj.Groups(1).Signals(1).XData = [0 60]
      | sbobj.Groups(1).Signals(1).YData = [0 0]
      | sbobj.Groups(1).Signals(2).Name = 'HULL'
      | sbobj.Groups(1).Signals(2).XData = [0 10.2 10.2 36 60]
      | sbobj.Groups(1).Signals(2).YData = [0 0 1 1 1]
      | sbobj.Groups(1).TimeRange = [0 60]
      | sbobj.Groups(2).Name = 'DISK_THEN_LOAD'
      | sbobj.Groups(2).Signals(1).Name = 'DISK'
      | sbobj.Groups(2).Signals(1).XData = [0 5 29.99 30 60]
      | sbobj.Groups(2).Signals(1).YData = [1 1 1 0 0]
      | sbobj.Groups(2).Signals(2).Name = 'HULL'
      | sbobj.Groups(2).Signals(2).XData = [0 10.2 10.2 36 60]
      | sbobj.Groups(2).Signals(2).YData = [0 0 1 1 1]
      | sbobj.Groups(2).TimeRange = [0 60]
      | sbobj.Groups(3).Name = 'LOAD_THEN_DISK'
      | sbobj.Groups(3).Signals(1).Name = 'DISK'
      | sbobj.Groups(3).Signals(1).XData = [0 10 10 30 30 60]
      | sbobj.Groups(3).Signals(1).YData = [0 0 1 1 0 0]
      | sbobj.Groups(3).Signals(2).Name = 'HULL'
      | sbobj.Groups(3).Signals(2).XData = [0 10.2 36 60]
      | sbobj.Groups(3).Signals(2).YData = [1 1 1 1]
      | sbobj.Groups(3).TimeRange = [0 60]
      | sbobj.Groups(4).Name = 'DISK_THEN_LOAD_V2'
      | sbobj.Groups(4).Signals(1).Name = 'DISK'
      | sbobj.Groups(4).Signals(1).XData = [0 5 20 60]
      | sbobj.Groups(4).Signals(1).YData = [1 1 1 1]
      | sbobj.Groups(4).Signals(2).Name = 'HULL'
      | sbobj.Groups(4).Signals(2).XData = [0 10.2 10.2 36 60]
      | sbobj.Groups(4).Signals(2).YData = [0 0 1 1 1]
      | sbobj.Groups(4).TimeRange = [0 60]
      | sbobj.Groups(5).Name = 'DISK_ON_AND_3_STEP_CHANGES'
      | sbobj.Groups(5).Signals(1).Name = 'DISK'
      | sbobj.Groups(5).Signals(1).XData = [0 5 20 20 30 30 40 40 60]
      | sbobj.Groups(5).Signals(1).YData = [1 1 1 0.7 0.7 0.4 0.4 1 1]
      | sbobj.Groups(5).Signals(2).Name = 'HULL'
      | sbobj.Groups(5).Signals(2).XData = [0 10.2 10.2 36 60]
      | sbobj.Groups(5).Signals(2).YData = [0 0 1 1 1]
      | sbobj.Groups(5).TimeRange = [0 60]
      | sbobj.Groups(6).Name = 'RAMP_TO_10PC'
      | sbobj.Groups(6).Signals(1).Name = 'DISK'
      | sbobj.Groups(6).Signals(1).XData = [0 60]
      | sbobj.Groups(6).Signals(1).YData = [1 0.1]
      | sbobj.Groups(6).Signals(2).Name = 'HULL'
      | sbobj.Groups(6).Signals(2).XData = [0 10.2 10.2 36 60]
      | sbobj.Groups(6).Signals(2).YData = [0 0 1 1 1]
      | sbobj.Groups(6).TimeRange = [0 60]
  DISK : Outport  Tag=STV Outport
  HULL : Outport  Tag=STV Outport  Port=2
  wires:
  FromWs/1 -> Demux/1
  Demux/1 -> DISK/1
  Demux/2 -> HULL/1

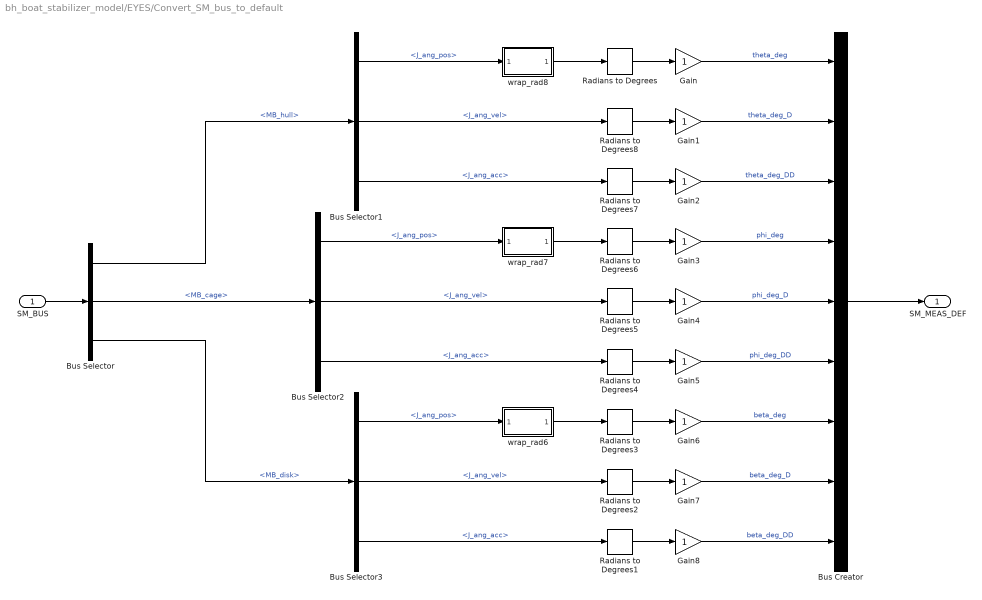
== system bh_boat_stabilizer_model/EYES/Convert_SM_bus_to_default ==
  SM_BUS : Inport
  Bus Creator : BusCreator  Inputs=9
  Bus Selector : BusSelector  OutputSignals=MB_hull,MB_cage,MB_disk
  Bus Selector1 : BusSelector  OutputSignals=J_ang_pos,J_ang_vel,J_ang_acc
  Bus Selector2 : BusSelector  OutputSignals=J_ang_pos,J_ang_vel,J_ang_acc
  Bus Selector3 : BusSelector  OutputSignals=J_ang_pos,J_ang_vel,J_ang_acc
  Gain{,1..8} (9 alike) : Gain
  Radians to Degrees{,1..8} (9 alike) : simulink_extras/Transformations/Radians to Degrees
  wrap_rad6 : Subsystem
  wrap_rad7 : Subsystem
  wrap_rad8 : Subsystem
  SM_MEAS_DEF : Outport
  wires:
  SM_BUS/1 -> Bus Selector/1
  Bus Selector/1 -> Bus Selector1/1  "<MB_hull>"
  Gain/1 -> Bus Creator/1  "theta_deg"
  Gain1/1 -> Bus Creator/2  "theta_deg_D"
  Gain2/1 -> Bus Creator/3  "theta_deg_DD"
  Gain4/1 -> Bus Creator/5  "phi_deg_D"
  Gain5/1 -> Bus Creator/6  "phi_deg_DD"
  Gain3/1 -> Bus Creator/4  "phi_deg"
  Gain7/1 -> Bus Creator/8  "beta_deg_D"
  Gain8/1 -> Bus Creator/9  "beta_deg_DD"
  Gain6/1 -> Bus Creator/7  "beta_deg"
  Bus Selector1/1 -> wrap_rad8/1(ang_radians)  "<J_ang_pos>"
  Bus Selector1/2 -> Radians to Degrees8/1  "<J_ang_vel>"
  Bus Selector1/3 -> Radians to Degrees7/1  "<J_ang_acc>"
  Bus Selector/2 -> Bus Selector2/1  "<MB_cage>"
  Bus Selector2/1 -> wrap_rad7/1(ang_radians)  "<J_ang_pos>"
  Bus Selector2/2 -> Radians to Degrees5/1  "<J_ang_vel>"
  Bus Selector2/3 -> Radians to Degrees4/1  "<J_ang_acc>"
  Bus Selector3/1 -> wrap_rad6/1(ang_radians)  "<J_ang_pos>"
  Bus Selector3/2 -> Radians to Degrees2/1  "<J_ang_vel>"
  Bus Selector3/3 -> Radians to Degrees1/1  "<J_ang_acc>"
  Bus Selector/3 -> Bus Selector3/1  "<MB_disk>"
  Bus Creator/1 -> SM_MEAS_DEF/1
  Radians to Degrees/1 -> Gain/1
  Radians to Degrees8/1 -> Gain1/1
  Radians to Degrees7/1 -> Gain2/1
  Radians to Degrees6/1 -> Gain3/1
  Radians to Degrees5/1 -> Gain4/1
  Radians to Degrees4/1 -> Gain5/1
  Radians to Degrees3/1 -> Gain6/1
  Radians to Degrees2/1 -> Gain7/1
  Radians to Degrees1/1 -> Gain8/1
  wrap_rad8/1(ang_wrapped) -> Radians to Degrees/1
  wrap_rad7/1(ang_wrapped) -> Radians to Degrees6/1
  wrap_rad6/1(ang_wrapped) -> Radians to Degrees3/1

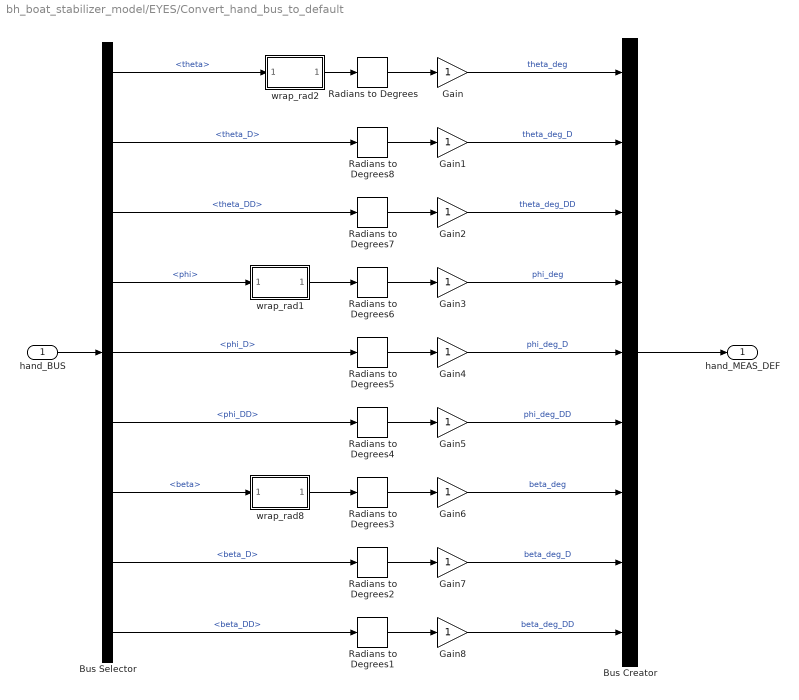
== system bh_boat_stabilizer_model/EYES/Convert_hand_bus_to_default ==
  hand_BUS : Inport
  Bus Creator : BusCreator  Inputs=9
  Bus Selector : BusSelector  OutputSignals=theta,theta_D,theta_DD,phi,phi_D,phi_DD,beta,beta_D,beta_DD
  Gain{,1..8} (9 alike) : Gain
  Radians to Degrees{,1..8} (9 alike) : simulink_extras/Transformations/Radians to Degrees
  wrap_rad1 : Subsystem
  wrap_rad2 : Subsystem
  wrap_rad8 : Subsystem
  hand_MEAS_DEF : Outport
  wires:
  Gain/1 -> Bus Creator/1  "theta_deg"
  Gain1/1 -> Bus Creator/2  "theta_deg_D"
  Gain2/1 -> Bus Creator/3  "theta_deg_DD"
  Gain4/1 -> Bus Creator/5  "phi_deg_D"
  Gain5/1 -> Bus Creator/6  "phi_deg_DD"
  Gain3/1 -> Bus Creator/4  "phi_deg"
  Gain7/1 -> Bus Creator/8  "beta_deg_D"
  Gain8/1 -> Bus Creator/9  "beta_deg_DD"
  Gain6/1 -> Bus Creator/7  "beta_deg"
  Bus Creator/1 -> hand_MEAS_DEF/1
  Radians to Degrees/1 -> Gain/1
  Radians to Degrees8/1 -> Gain1/1
  Radians to Degrees7/1 -> Gain2/1
  Radians to Degrees6/1 -> Gain3/1
  Radians to Degrees5/1 -> Gain4/1
  Radians to Degrees4/1 -> Gain5/1
  Radians to Degrees3/1 -> Gain6/1
  Radians to Degrees2/1 -> Gain7/1
  Radians to Degrees1/1 -> Gain8/1
  Bus Selector/1 -> wrap_rad2/1(ang_radians)  "<theta>"
  Bus Selector/4 -> wrap_rad1/1(ang_radians)  "<phi>"
  Bus Selector/7 -> wrap_rad8/1(ang_radians)  "<beta>"
  hand_BUS/1 -> Bus Selector/1
  Bus Selector/9 -> Radians to Degrees1/1  "<beta_DD>"
  Bus Selector/8 -> Radians to Degrees2/1  "<beta_D>"
  Bus Selector/6 -> Radians to Degrees4/1  "<phi_DD>"
  Bus Selector/5 -> Radians to Degrees5/1  "<phi_D>"
  Bus Selector/3 -> Radians to Degrees7/1  "<theta_DD>"
  Bus Selector/2 -> Radians to Degrees8/1  "<theta_D>"
  wrap_rad2/1(ang_wrapped) -> Radians to Degrees/1
  wrap_rad1/1(ang_wrapped) -> Radians to Degrees6/1
  wrap_rad8/1(ang_wrapped) -> Radians to Degrees3/1

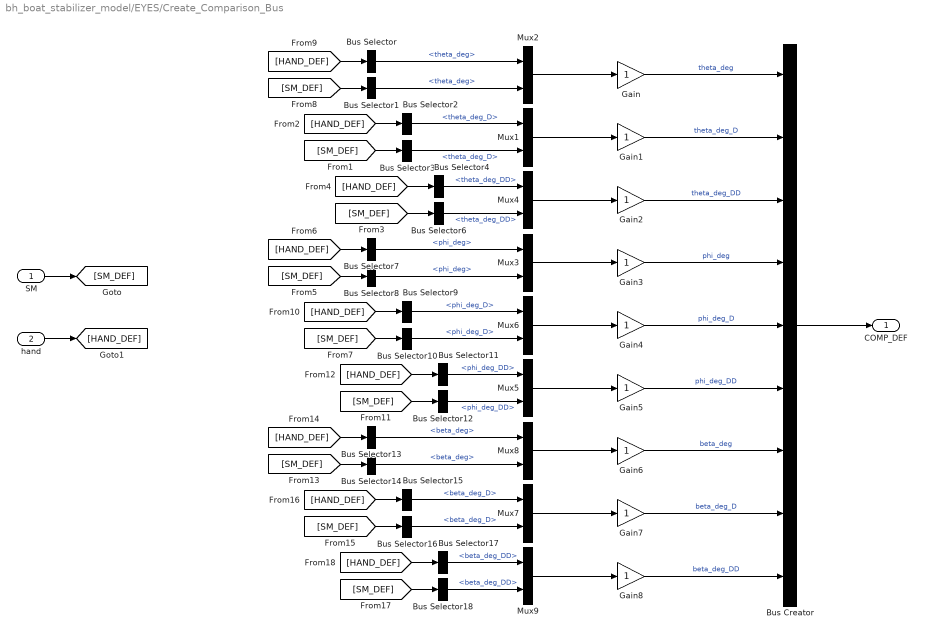
== system bh_boat_stabilizer_model/EYES/Create_Comparison_Bus ==
  SM : Inport
  hand : Inport  Port=2
  Bus Creator : BusCreator  Inputs=9
  Bus Selector : BusSelector  OutputSignals=theta_deg
  Bus Selector1 : BusSelector  OutputSignals=theta_deg
  Bus Selector10 : BusSelector  OutputSignals=phi_deg_D
  Bus Selector11 : BusSelector  OutputSignals=phi_deg_DD
  Bus Selector12 : BusSelector  OutputSignals=phi_deg_DD
  Bus Selector13 : BusSelector  OutputSignals=beta_deg
  Bus Selector14 : BusSelector  OutputSignals=beta_deg
  Bus Selector15 : BusSelector  OutputSignals=beta_deg_D
  Bus Selector16 : BusSelector  OutputSignals=beta_deg_D
  Bus Selector17 : BusSelector  OutputSignals=beta_deg_DD
  Bus Selector18 : BusSelector  OutputSignals=beta_deg_DD
  Bus Selector2 : BusSelector  OutputSignals=theta_deg_D
  Bus Selector3 : BusSelector  OutputSignals=theta_deg_D
  Bus Selector4 : BusSelector  OutputSignals=theta_deg_DD
  Bus Selector6 : BusSelector  OutputSignals=theta_deg_DD
  Bus Selector7 : BusSelector  OutputSignals=phi_deg
  Bus Selector8 : BusSelector  OutputSignals=phi_deg
  Bus Selector9 : BusSelector  OutputSignals=phi_deg_D
  Gain{,1..8} (9 alike) : Gain
  Mux{1..9} (9 alike) : Mux  Inputs=2
  COMP_DEF : Outport
  wires:
  hand/1 -> [HAND_DEF]
  SM/1 -> [SM_DEF]
  Gain5/1 -> Bus Creator/6  "phi_deg_DD"
  Gain4/1 -> Bus Creator/5  "phi_deg_D"
  Gain/1 -> Bus Creator/1  "theta_deg"
  Gain2/1 -> Bus Creator/3  "theta_deg_DD"
  Bus Creator/1 -> COMP_DEF/1
  Gain6/1 -> Bus Creator/7  "beta_deg"
  Gain1/1 -> Bus Creator/2  "theta_deg_D"
  Gain8/1 -> Bus Creator/9  "beta_deg_DD"
  Gain3/1 -> Bus Creator/4  "phi_deg"
  Gain7/1 -> Bus Creator/8  "beta_deg_D"
  Mux2/1 -> Gain/1
  Mux1/1 -> Gain1/1
  Mux3/1 -> Gain3/1
  Mux4/1 -> Gain2/1
  Mux8/1 -> Gain6/1
  Mux5/1 -> Gain5/1
  Mux7/1 -> Gain7/1
  Mux6/1 -> Gain4/1
  Mux9/1 -> Gain8/1
  [HAND_DEF] -> Bus Selector/1
  [SM_DEF] -> Bus Selector1/1
  Bus Selector/1 -> Mux2/1  "<theta_deg>"
  Bus Selector1/1 -> Mux2/2  "<theta_deg>"
  [SM_DEF] -> Bus Selector3/1
  Bus Selector3/1 -> Mux1/2  "<theta_deg_D>"
  Bus Selector2/1 -> Mux1/1  "<theta_deg_D>"
  [HAND_DEF] -> Bus Selector2/1
  [SM_DEF] -> Bus Selector6/1
  Bus Selector6/1 -> Mux4/2  "<theta_deg_DD>"
  Bus Selector4/1 -> Mux4/1  "<theta_deg_DD>"
  [HAND_DEF] -> Bus Selector4/1
  [SM_DEF] -> Bus Selector8/1
  Bus Selector8/1 -> Mux3/2  "<phi_deg>"
  Bus Selector7/1 -> Mux3/1  "<phi_deg>"
  [HAND_DEF] -> Bus Selector7/1
  [SM_DEF] -> Bus Selector10/1
  Bus Selector10/1 -> Mux6/2  "<phi_deg_D>"
  Bus Selector9/1 -> Mux6/1  "<phi_deg_D>"
  [HAND_DEF] -> Bus Selector9/1
  [SM_DEF] -> Bus Selector12/1
  Bus Selector12/1 -> Mux5/2  "<phi_deg_DD>"
  Bus Selector11/1 -> Mux5/1  "<phi_deg_DD>"
  [HAND_DEF] -> Bus Selector11/1
  [SM_DEF] -> Bus Selector14/1
  Bus Selector14/1 -> Mux8/2  "<beta_deg>"
  Bus Selector13/1 -> Mux8/1  "<beta_deg>"
  [HAND_DEF] -> Bus Selector13/1
  [SM_DEF] -> Bus Selector16/1
  Bus Selector16/1 -> Mux7/2  "<beta_deg_D>"
  Bus Selector15/1 -> Mux7/1  "<beta_deg_D>"
  [HAND_DEF] -> Bus Selector15/1
  [SM_DEF] -> Bus Selector18/1
  Bus Selector18/1 -> Mux9/2  "<beta_deg_DD>"
  Bus Selector17/1 -> Mux9/1  "<beta_deg_DD>"
  [HAND_DEF] -> Bus Selector17/1

== system bh_boat_stabilizer_model/Boat_plant_Simscape/Boat_SM/Check_CoMs ==
  PS-Simulink Converter6 : nesl_utility/PS-Simulink Converter  PhysicalDomain=network_engine_domain  SubClassName=ps_output  LeftPortType=input  RightPortType=output  PseudoPeriodic=off  Frequencies=[]  VectorFormat=1-D array  Unit=m  AffineConversion=off
  PS-Simulink Converter7 : nesl_utility/PS-Simulink Converter  PhysicalDomain=network_engine_domain  SubClassName=ps_output  LeftPortType=input  RightPortType=output  PseudoPeriodic=off  Frequencies=[]  VectorFormat=1-D array  Unit=m  AffineConversion=off
  PS-Simulink Converter8 : nesl_utility/PS-Simulink Converter  PhysicalDomain=network_engine_domain  SubClassName=ps_output  LeftPortType=input  RightPortType=output  PseudoPeriodic=off  Frequencies=[]  VectorFormat=1-D array  Unit=m  AffineConversion=off
  Scope2 : Scope  NumInputPorts=3
  Transform Sensor2 : sm_lib/Frames and Transforms/Transform Sensor  MeasurementFrame=Base  SenseAngle=off  SenseAxis=off  SenseQ=off  SenseR=off  SenseRotationSequence=off  RotationSequence=XYX  SenseOmegaX=off  SenseOmegaY=off  SenseOmegaZ=off  SenseQDot=off  SenseRDot=off  SenseAlphaX=off  SenseAlphaY=off  SenseAlphaZ=off  SenseQDDot=off  SenseRDDot=off  SenseX=on  SenseY=on  SenseZ=on  SenseRad=off  SenseAzim=off  SenseDist=off  SenseInc=off  SenseXDot=off  SenseYDot=off  SenseZDot=off  SenseRadDot=off  SenseAzimDot=off  SenseDistDot=off  SenseIncDot=off  SenseXDDot=off  SenseYDDot=off  SenseZDDot=off  SenseRadDDot=off  SenseAzimDDot=off  SenseDistDDot=off  SenseIncDDot=off
  F : PMIOPort  Side=Left
  O_H : PMIOPort  Port=2  Side=Right
  wires:
  PS-Simulink Converter7/1 -> Scope2/2
  PS-Simulink Converter6/1 -> Scope2/1
  PS-Simulink Converter8/1 -> Scope2/3
  connections:
  PS-Simulink Converter6/LConn1 -- Transform Sensor2/RConn2
  Transform Sensor2/RConn4 -- PS-Simulink Converter8/LConn1
  Transform Sensor2/RConn3 -- PS-Simulink Converter7/LConn1
  O_H/RConn1 -- Transform Sensor2/LConn1
  F/RConn1 -- Transform Sensor2/RConn1

== system bh_boat_stabilizer_model/Boat_plant_Simscape/Boat_SM/Check_CoMs1 ==
  PS-Simulink Converter6 : nesl_utility/PS-Simulink Converter  PhysicalDomain=network_engine_domain  SubClassName=ps_output  LeftPortType=input  RightPortType=output  PseudoPeriodic=off  Frequencies=[]  VectorFormat=1-D array  Unit=m  AffineConversion=off
  PS-Simulink Converter7 : nesl_utility/PS-Simulink Converter  PhysicalDomain=network_engine_domain  SubClassName=ps_output  LeftPortType=input  RightPortType=output  PseudoPeriodic=off  Frequencies=[]  VectorFormat=1-D array  Unit=m  AffineConversion=off
  PS-Simulink Converter8 : nesl_utility/PS-Simulink Converter  PhysicalDomain=network_engine_domain  SubClassName=ps_output  LeftPortType=input  RightPortType=output  PseudoPeriodic=off  Frequencies=[]  VectorFormat=1-D array  Unit=m  AffineConversion=off
  Scope2 : Scope  NumInputPorts=3
  Transform Sensor2 : sm_lib/Frames and Transforms/Transform Sensor  MeasurementFrame=Base  SenseAngle=off  SenseAxis=off  SenseQ=off  SenseR=off  SenseRotationSequence=off  RotationSequence=XYX  SenseOmegaX=off  SenseOmegaY=off  SenseOmegaZ=off  SenseQDot=off  SenseRDot=off  SenseAlphaX=off  SenseAlphaY=off  SenseAlphaZ=off  SenseQDDot=off  SenseRDDot=off  SenseX=on  SenseY=on  SenseZ=on  SenseRad=off  SenseAzim=off  SenseDist=off  SenseInc=off  SenseXDot=off  SenseYDot=off  SenseZDot=off  SenseRadDot=off  SenseAzimDot=off  SenseDistDot=off  SenseIncDot=off  SenseXDDot=off  SenseYDDot=off  SenseZDDot=off  SenseRadDDot=off  SenseAzimDDot=off  SenseDistDDot=off  SenseIncDDot=off
  F : PMIOPort  Side=Left
  O_H : PMIOPort  Port=2  Side=Right
  wires:
  PS-Simulink Converter7/1 -> Scope2/2
  PS-Simulink Converter6/1 -> Scope2/1
  PS-Simulink Converter8/1 -> Scope2/3
  connections:
  PS-Simulink Converter6/LConn1 -- Transform Sensor2/RConn2
  Transform Sensor2/RConn4 -- PS-Simulink Converter8/LConn1
  Transform Sensor2/RConn3 -- PS-Simulink Converter7/LConn1
  O_H/RConn1 -- Transform Sensor2/LConn1
  F/RConn1 -- Transform Sensor2/RConn1

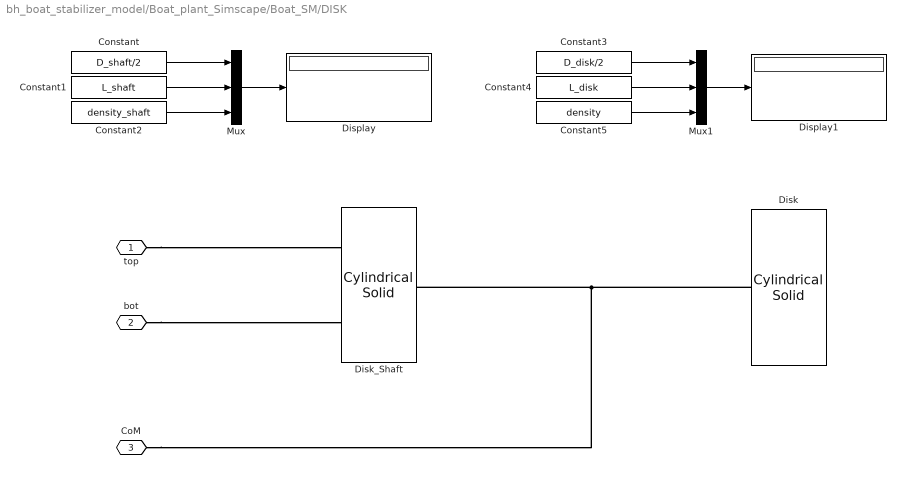
== system bh_boat_stabilizer_model/Boat_plant_Simscape/Boat_SM/DISK ==
  Constant : Constant  Value=D_shaft/2
  Constant1 : Constant  Value=L_shaft
  Constant2 : Constant  Value=density_shaft
  Constant3 : Constant  Value=D_disk/2
  Constant4 : Constant  Value=L_disk
  Constant5 : Constant  Value=density
  Disk : sm_lib/Body Elements/Cylindrical Solid  GraphicAmbientColor=[0.15 0.15 0.15 1.0]  BasedOnType=Density  CenterOfMass=[0 0 0]  CenterOfMassUnits=m  GraphicDiffuseColor=[1.0 1.0 0.0]  CylinderLength=L_disk  CylinderLengthUnits=m  CylinderRadius=D_disk/2  CylinderRadiusUnits=m  Density=density  DensityUnits=kg/m^3  DoExposeReferenceFrame=on  GraphicEmissiveColor=[0.0 0.0 0.0 1.0]  ExportEntireGeometry=off  SerializedFrames=<Frames/>  MarkerShape=Sphere  MarkerSize=10  GraphicType=FromGeometry  InertiaType=CalculateFromGeometry  Mass=1  MassUnits=kg  MomentsOfInertia=[1 1 1]  MomentsOfInertiaUnits=kg*m^2  GraphicOpacity=1.0  ProductsOfInertia=[0 0 0]  ProductsOfInertiaUnits=kg*m^2  GraphicShininess=75  GraphicSpecularColor=[0.5 0.5 0.5 1.0]  GraphicVisPropType=SimpleVisualProperties
      settings: AttributesFormatString=|
      | Radius = %<CylinderRadius> (%<CylinderRadiusUnits>)
      | L = %<CylinderLength> (%<CylinderLengthUnits>)
      | Density = %<Density>(%<DensityUnits>)
  Disk_Shaft : sm_lib/Body Elements/Cylindrical Solid  GraphicAmbientColor=[0.15 0.15 0.15 1.0]  BasedOnType=Density  CenterOfMass=[0 0 0]  CenterOfMassUnits=m  GraphicDiffuseColor=[1.0 1.0 0.0]  CylinderLength=L_shaft  CylinderLengthUnits=m  CylinderRadius=D_shaft/2  CylinderRadiusUnits=m  Density=density_shaft  DensityUnits=kg/m^3  DoExposeReferenceFrame=on  GraphicEmissiveColor=[0.0 0.0 0.0 1.0]  ExportEntireGeometry=off  SerializedFrames=<Frames><Frame><Id>Frame1</Id><Value><Name>Top</Name><Origin><Source>GeometricFeature</Source><FeatureName>top surface</FeatureName></Origin><PrimaryAxis><DefinedDirection>+Z</DefinedDirection><Source>ReferenceFrame</Source><SourceDirection>+Z</SourceDirection><FeatureName></FeatureName></PrimaryAxis><SecondaryAxis><DefinedDirection>+X</DefinedDirection><Source>ReferenceFrame</Source><SourceDirection>+X</SourceDirection><FeatureName></FeatureName></SecondaryAxis></Value></Frame><Frame><Id>Frame2</Id><Value><Name>Bot</Name><Origin><Source>GeometricFeature</Source><FeatureName>bottom surface</FeatureName></Origin><PrimaryAxis><DefinedDirection>+Z</DefinedDirection><Source>ReferenceFrame</Source><SourceDirection>+Z</SourceDirection><FeatureName></FeatureName></PrimaryAxis><SecondaryAxis><DefinedDirection>+X</DefinedDirection><Source>ReferenceFrame</Source><SourceDirection>+X</SourceDirection><FeatureName></FeatureName></SecondaryAxis></Value></Frame></Frames>  MarkerShape=Sphere  MarkerSize=10  GraphicType=FromGeometry  InertiaType=CalculateFromGeometry  Mass=1  MassUnits=kg  MomentsOfInertia=[1 1 1]  MomentsOfInertiaUnits=kg*m^2  GraphicOpacity=1.0  ProductsOfInertia=[0 0 0]  ProductsOfInertiaUnits=kg*m^2  GraphicShininess=75  GraphicSpecularColor=[0.5 0.5 0.5 1.0]  GraphicVisPropType=SimpleVisualProperties
      settings: AttributesFormatString=|
      | Radius = %<CylinderRadius> (%<CylinderRadiusUnits>)
      | L = %<CylinderLength> (%<CylinderLengthUnits>)
      | Density = %<Density>(%<DensityUnits>)
  Display : Display
  Display1 : Display
  Mux : Mux  Inputs=3
  Mux1 : Mux  Inputs=3
  top : PMIOPort  Side=Right
  bot : PMIOPort  Port=2  Side=Left
  CoM : PMIOPort  Port=3  Side=Left
  wires:
  Mux/1 -> Display/1
  Constant/1 -> Mux/1
  Constant2/1 -> Mux/3
  Constant1/1 -> Mux/2
  Constant3/1 -> Mux1/1
  Constant4/1 -> Mux1/2
  Constant5/1 -> Mux1/3
  Mux1/1 -> Display1/1
  connections:
  bot/RConn1 -- Disk_Shaft/LConn2
  top/RConn1 -- Disk_Shaft/LConn1
  Disk/RConn1 -- CoM/RConn1 -- Disk_Shaft/RConn1
